simulink model "AttitudeProcessingANDStateEstimator"  (R2017b)
settings: Solver=FixedStepAuto  StartTime=0.0  StopTime=10.0  FixedStep=0.08  RelTol=1e-3
libraries: MATLAB_Function_lib x7, simulink x2
settings Model: Creator=hbourbou  LastModifiedBy=hbourbou
settings ModelReferenceCC: ModelReferenceNumInstancesAllowed=Single

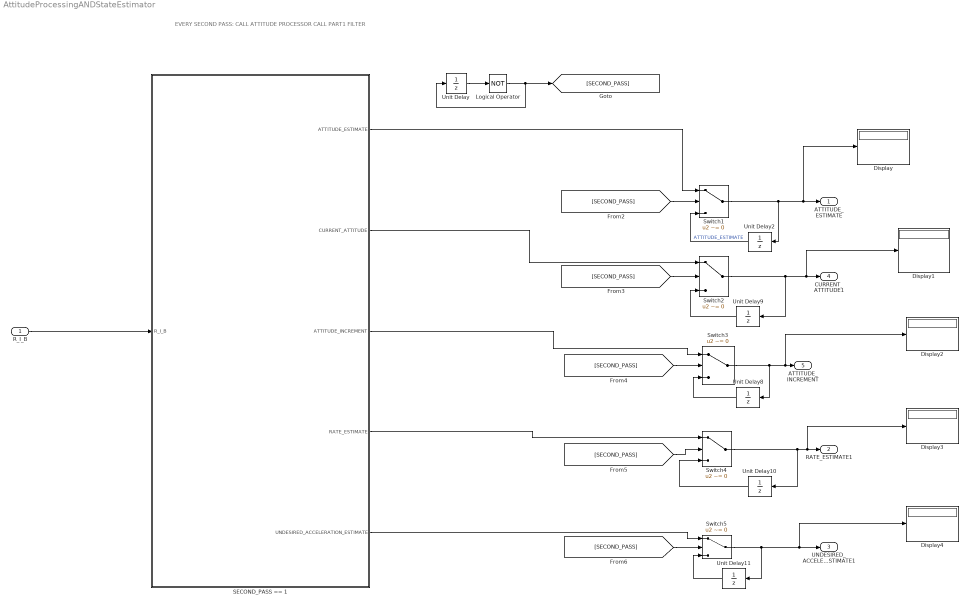
== system AttitudeProcessingANDStateEstimator ==
  note: EVERY SECOND PASS:
      | CALL ATTITUDE PROCESSOR
      | CALL PART1 FILTER
  R_I_B : Inport
  Display{,1..4} (5 alike) : Display
  Logical Operator : Logic  Operator=NOT  Inputs=1  AllPortsSameDT=off  OutDataTypeStr=boolean
  SECOND_PASS == 1 : Subsystem  TreatAsAtomicUnit=on
  Switch{1..5} (5 alike) : Switch  Criteria=u2 ~= 0
  Unit Delay : UnitDelay  InitialCondition=false  SampleTime=-1
  Unit Delay10 : UnitDelay  InitialCondition=[-13.09;0;0]  SampleTime=-1
  Unit Delay11 : UnitDelay  InitialCondition=[-163.6;0;0]  SampleTime=-1
  Unit Delay2 : UnitDelay  InitialCondition=[-1;0;0]  SampleTime=-1
  Unit Delay8 : UnitDelay  InitialCondition=[-1;0;0]  SampleTime=-1
  Unit Delay9 : UnitDelay  InitialCondition=[0;0.5;0;0]  SampleTime=-1
  ATTITUDE_ESTIMATE : Outport
  RATE_ESTIMATE1 : Outport  Port=2
  UNDESIRED_ACCELERATION_ESTIMATE1 : Outport  Port=3
  CURRENT_ATTITUDE1 : Outport  Port=4
  ATTITUDE_INCREMENT : Outport  Port=5
  wires:
  SECOND_PASS == 1/2(CURRENT_ATTITUDE) -> Switch2/1
  Logical Operator/1 -> [SECOND_PASS], Unit Delay/1
  SECOND_PASS == 1/5(UNDESIRED_ACCELERATION_ESTIMATE) -> Switch5/1
  SECOND_PASS == 1/4(RATE_ESTIMATE) -> Switch4/1
  Unit Delay10/1 -> Switch4/3
  SECOND_PASS == 1/3(ATTITUDE_INCREMENT) -> Switch3/1
  Unit Delay8/1 -> Switch3/3
  Unit Delay11/1 -> Switch5/3
  Switch2/1 -> Unit Delay9/1, Display1/1, CURRENT_ATTITUDE1/1
  Unit Delay9/1 -> Switch2/3
  Switch3/1 -> Display2/1, ATTITUDE_INCREMENT/1, Unit Delay8/1
  SECOND_PASS == 1/1(ATTITUDE_ESTIMATE) -> Switch1/1
  R_I_B/1 -> SECOND_PASS == 1/1(R_I_B)
  Switch4/1 -> Unit Delay10/1, Display3/1, RATE_ESTIMATE1/1
  Switch5/1 -> Unit Delay11/1, Display4/1, UNDESIRED_ACCELERATION_ESTIMATE1/1
  [SECOND_PASS] -> Switch1/2
  [SECOND_PASS] -> Switch2/2
  [SECOND_PASS] -> Switch3/2
  [SECOND_PASS] -> Switch4/2
  [SECOND_PASS] -> Switch5/2
  Switch1/1 -> Unit Delay2/1, Display/1, ATTITUDE_ESTIMATE/1
  Unit Delay2/1 -> Switch1/3  "ATTITUDE_ESTIMATE"
  Unit Delay/1 -> Logical Operator/1

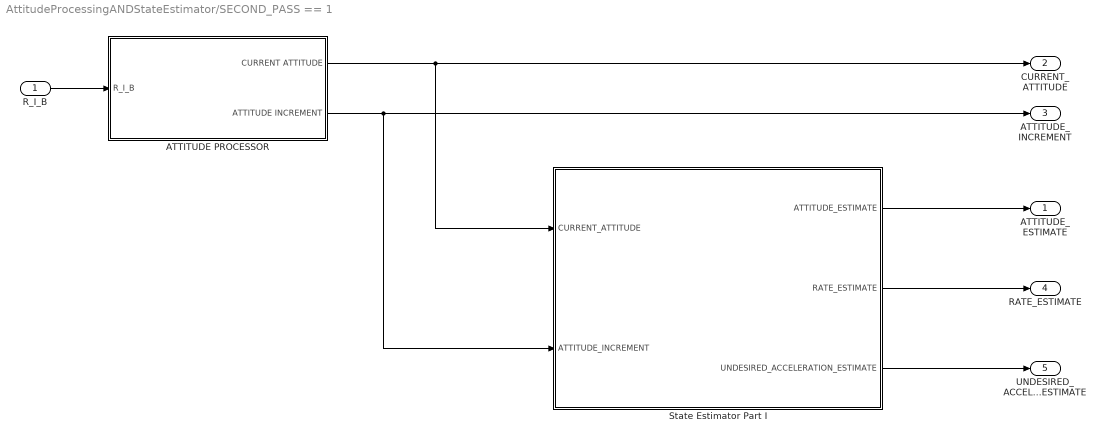
== system AttitudeProcessingANDStateEstimator/SECOND_PASS == 1 ==
  R_I_B : Inport
  ATTITUDE PROCESSOR : Subsystem
  State Estimator Part I : Subsystem
  ATTITUDE_ESTIMATE : Outport
  CURRENT_ATTITUDE : Outport  Port=2
  ATTITUDE_INCREMENT : Outport  Port=3
  RATE_ESTIMATE : Outport  Port=4
  UNDESIRED_ACCELERATION_ESTIMATE : Outport  Port=5
  wires:
  ATTITUDE PROCESSOR/2(ATTITUDE INCREMENT) -> State Estimator Part I/2(ATTITUDE_INCREMENT), ATTITUDE_INCREMENT/1
  R_I_B/1 -> ATTITUDE PROCESSOR/1(R_I_B)
  State Estimator Part I/1(ATTITUDE_ESTIMATE) -> ATTITUDE_ESTIMATE/1
  State Estimator Part I/2(RATE_ESTIMATE) -> RATE_ESTIMATE/1
  State Estimator Part I/3(UNDESIRED_ACCELERATION_ESTIMATE) -> UNDESIRED_ACCELERATION_ESTIMATE/1
  ATTITUDE PROCESSOR/1(CURRENT ATTITUDE) -> State Estimator Part I/1(CURRENT_ATTITUDE), CURRENT_ATTITUDE/1

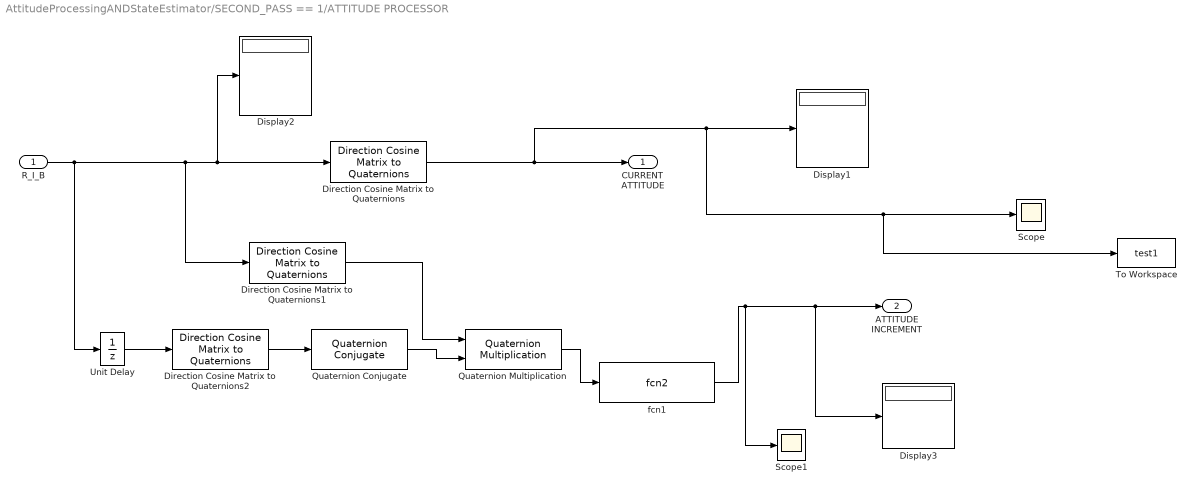
== system AttitudeProcessingANDStateEstimator/SECOND_PASS == 1/ATTITUDE PROCESSOR ==
  R_I_B : Inport
  Direction Cosine Matrix to Quaternions : MATLAB_Function_lib/Direction Cosine Matrix  to Quaternions
  Direction Cosine Matrix to Quaternions1 : MATLAB_Function_lib/Direction Cosine Matrix  to Quaternions
  Direction Cosine Matrix to Quaternions2 : MATLAB_Function_lib/Direction Cosine Matrix  to Quaternions
  Display1 : Display
  Display2 : Display
  Display3 : Display
  Quaternion Conjugate : MATLAB_Function_lib/Quaternion Conjugate
  Quaternion Multiplication : MATLAB_Function_lib/Quaternion Multiplication
  Scope : Scope
  Scope1 : Scope
  To Workspace : ToWorkspace  VariableName=test1  SaveFormat=Timeseries  SampleTime=-1
  Unit Delay : UnitDelay  InitialCondition=eye(3)  SampleTime=-1
  fcn1 : MATLAB_Function_lib/fcn2
  CURRENT ATTITUDE : Outport
  ATTITUDE INCREMENT : Outport  Port=2
  wires:
  R_I_B/1 -> Direction Cosine Matrix to Quaternions1/1, Display2/1, Direction Cosine Matrix to Quaternions/1, Unit Delay/1
  Direction Cosine Matrix to Quaternions/1 -> To Workspace/1, Scope/1, Display1/1, CURRENT ATTITUDE/1
  fcn1/1 -> Scope1/1, Display3/1, ATTITUDE INCREMENT/1
  Direction Cosine Matrix to Quaternions2/1 -> Quaternion Conjugate/1
  Direction Cosine Matrix to Quaternions1/1 -> Quaternion Multiplication/1
  Quaternion Conjugate/1 -> Quaternion Multiplication/2
  Quaternion Multiplication/1 -> fcn1/1
  Unit Delay/1 -> Direction Cosine Matrix to Quaternions2/1

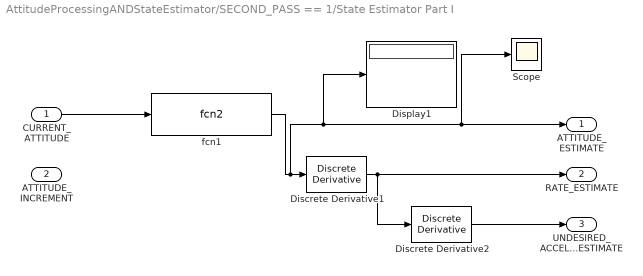
== system AttitudeProcessingANDStateEstimator/SECOND_PASS == 1/State Estimator Part I ==
  CURRENT_ATTITUDE : Inport
  ATTITUDE_INCREMENT : Inport  Port=2
  Discrete Derivative1 : simulink/Discrete/Discrete Derivative  gainval=1.0  ICPrevScaledInput=0.0  OutMin=[]  OutMax=[]  OutDataType=fixdt(1, 16)  OutScaling=2^-10  DoSatur=off
  Discrete Derivative2 : simulink/Discrete/Discrete Derivative  gainval=1.0  ICPrevScaledInput=0.0  OutMin=[]  OutMax=[]  OutDataType=fixdt(1, 16)  OutScaling=2^-10  DoSatur=off
  Display1 : Display
  Scope : Scope
  fcn1 : MATLAB_Function_lib/fcn2
  ATTITUDE_ESTIMATE : Outport
  RATE_ESTIMATE : Outport  Port=2
  UNDESIRED_ACCELERATION_ESTIMATE : Outport  Port=3
  wires:
  Discrete Derivative1/1 -> Discrete Derivative2/1, RATE_ESTIMATE/1
  Discrete Derivative2/1 -> UNDESIRED_ACCELERATION_ESTIMATE/1
  CURRENT_ATTITUDE/1 -> fcn1/1
  fcn1/1 -> Discrete Derivative1/1, Display1/1, Scope/1, ATTITUDE_ESTIMATE/1
